simulink model "lookuptable"  (R2020a)
settings: Solver=FixedStepDiscrete  StartTime=0.0  StopTime=options.T_train  RelTol=1e-3
PreLoadFcn:
  | Ts = 0.1;
  | Plant = c2d(zpk([],[-1 -3 -5],1),Ts);
  | C0 = pid(1,1,1,'Ts',Ts,'IF','B','DF','B'); % define PID structure
  | C = pidtune(Plant,C0); % design PID
  | [Kp Ki Kd] = piddata(C); % obtain PID gains
  | FIS = sugfis;
  | FIS = addInput(FIS,[-10 10],'Name','E');
  | FIS = addMF(FIS,'E','gaussmf',[7 -10],'Name','Negative');
  | FIS = addMF(FIS,'E','gaussmf',[7 10],'Name','Positive');
  | FIS = addInput(FIS,[-10 10],'Name','CE');
  | FIS = addMF(FIS,'CE','gaussmf',[7 -10],'Name','Negative');
  | FIS = addMF(FIS,'CE','gaussmf',[7 10],'Name','Positive');
  | FIS = addOutput(FIS,[-20 20],'Name','u');
  | FIS = addMF(FIS,'u','constant',-20,'Name','Min');
  | FIS = addMF(FIS,'u','constant',0,'Name','Zero');
  | FIS = addMF(FIS,'u','constant',20,'Name','Max');
  | ruleList = [1 1 1 1 1;...   % Rule 1
  |             1 2 2 1 1;...   % Rule 2
  |             2 1 2 1 1;...   % Rule 3
  |             2 2 3 1 1];     % Rule 4
  | FIS = addRule(FIS,ruleList);GE = 10;
  | GCE = GE*(Kp-sqrt(Kp^2-4*Ki*Kd))/2/Ki;
  | GCU = Ki/GE;
  | GU = Kd/GCE;
  | Step = 1; % use 21 break points for both E and CE inputs
  | E = -10:Step:10;
  | CE = -10:Step:10;
  | N = length(E);
  | LookUpTableData = zeros(N);
  | for i=1:N
  |    for j=1:N
  |       % compute output u for each combination of break points
  |       LookUpTableData(i,j) = evalfis(FIS,[E(i) CE(j)]);
  |    end
  | end
undefined symbols (not defined in the file or in its folder): DiscIntNeverNeededParam, options
libraries: simulink x2, cstblocks x1
CloseFcn:
  | clear C E GCU Kd LookUpTableData Step j C0 FIS GE Ki N Ts ruleList CE GCE GU Kp Plant i
settings Model: FPTRunName=Active  Creator=The MathWorks, Inc.  LastModifiedBy=kekatos
settings DataIOCC: LimitDataPoints=on  SaveFormat=Array  ReturnWorkspaceOutputs=off
settings OptimizationCC: ExpressionDepthLimit=2147483647  LifeSpan=inf
settings DebuggingCC: UnderspecifiedInitializationDetection=Classic  MergeDetectMultiDrivingBlocksExec=none  SolverPrmCheckMsg=warning  FcnCallInpInsideContextMsg=warning  StateNameClashWarn=warning  SFUnexpectedBacktrackingDiag=warning  SFNoUnconditionalDefaultTransitionDiag=warning  SFExecutionAtInitializationDiag=none  ArithmeticOperatorsInVariantConditions=warning
settings HardwareCC: ProdBitPerPointer=32  ProdBitPerSizeT=32  ProdBitPerPtrDiffT=32  ProdLargestAtomicFloat=None  ProdIntDivRoundTo=Undefined  ProdEndianess=Unspecified  ProdWordSize=32  ProdHWDeviceType=32-bit Generic
settings ModelReferenceCC: PropagateSignalLabelsOutOfModel=off
settings SFSimCC: SimUseLocalCustomCode=off  CustomCodeUndefinedFunction=UseInterfaceOnly
settings RTWCC: RTWUseLocalCustomCode=off
settings CodeAppCC: StateflowObjectComments=on
settings GRTTargetCC: TargetLangStandard=C89/C90 (ANSI)  CombineOutputUpdateFcns=off  GRTInterface=on
settings ConfigComp: CovMetricSettings=dw  CovHtmlReporting=on  CovSaveCumulativeToWorkspaceVar=on  CovSaveSingleToWorkspaceVar=on  CovExternalEMLEnable=off

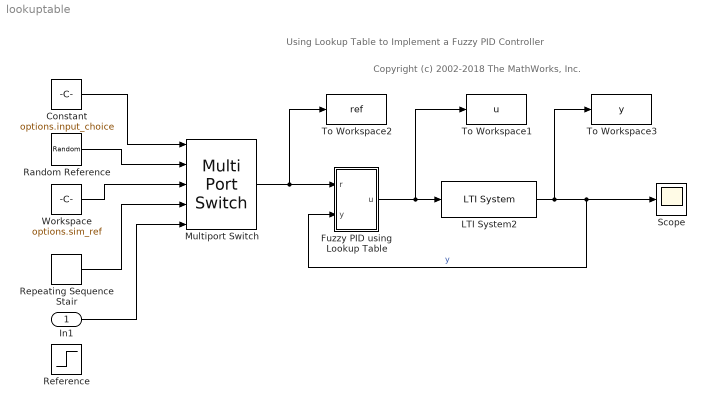
== system lookuptable ==
  note: Using Lookup Table to Implement a Fuzzy PID Controller
  note: Copyright (c) 2002-2018 The MathWorks, Inc.
  In1 : Inport
  Constant : Constant  Value=options.input_choice
  Fuzzy PID using Lookup Table : Subsystem
  LTI System2 : cstblocks/LTI System  sys=Plant  IC=[]
  Multiport Switch : MultiPortSwitch  Inputs=4
  Random Reference : UniformRandomNumber  Minimum=options.ref_min  Maximum=options.ref_max  Seed=randi(2^32,[1 ])  SampleTime=options.ref_Ts
  Reference : Step  SampleTime=0
  Repeating Sequence Stair : simulink/Sources/Repeating Sequence Stair  OutValues=options.sim_cov  tsamp=options.ref_Ts  OutMin=[]  OutMax=[]  OutDataTypeStr=double  OutputDataTypeScalingMode=double  OutDataType=fixdt(0,8)  ConRadixGroup=Best Precision: Vector-wise  OutScaling=2^-12
  Scope : Scope
  To Workspace1 : ToWorkspace  VariableName=u  SaveFormat=Structure With Time  SampleTime=options.dt
  To Workspace2 : ToWorkspace  VariableName=ref  SaveFormat=Structure With Time  SampleTime=options.dt
  To Workspace3 : ToWorkspace  VariableName=y  SaveFormat=Structure With Time  SampleTime=options.dt
  Workspace : Constant  Value=options.sim_ref
  wires:
  Fuzzy PID using Lookup Table/1(u) -> LTI System2/1, To Workspace1/1
  LTI System2/1 -> Scope/1, Fuzzy PID using Lookup Table/2(y), To Workspace3/1  "y"
  Workspace/1 -> Multiport Switch/3
  Random Reference/1 -> Multiport Switch/2
  Repeating Sequence Stair/1 -> Multiport Switch/4
  Constant/1 -> Multiport Switch/1
  In1/1 -> Multiport Switch/5
  Multiport Switch/1 -> To Workspace2/1, Fuzzy PID using Lookup Table/1(r)

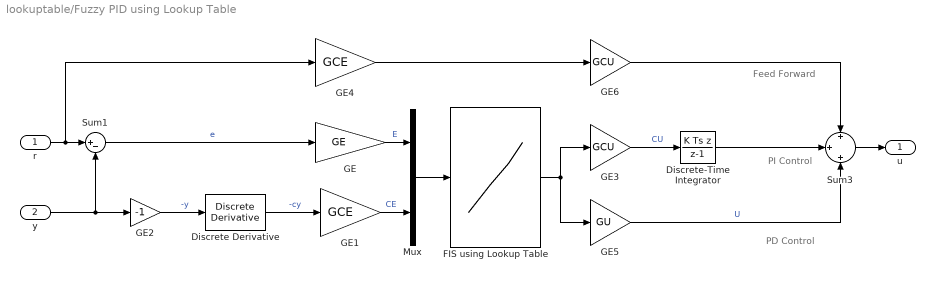
== system lookuptable/Fuzzy PID using Lookup Table ==
  note: PI Control
  note: PD Control
  note: Feed Forward
  r : Inport
  y : Inport  Port=2
  Discrete Derivative : simulink/Discrete/Discrete Derivative  gainval=1  ICPrevScaledInput=0.0  OutMin=[]  OutMax=[]  OutDataType=fixdt(1, 16)  OutScaling=2^-10  DoSatur=off
  Discrete-Time Integrator : DiscreteIntegrator  IntegratorMethod=Integration: Backward Euler  SampleTime=Ts  ICPrevOutput=DiscIntNeverNeededParam  ICPrevScaledInput=DiscIntNeverNeededParam
  FIS using Lookup Table : Lookup_n-D  BreakpointsForDimension1=E  BreakpointsForDimension2=CE  UseOneInputPortForAllInputData=on  Table=LookUpTableData  RndMeth=Simplest  InputSameDT=on
  GE : Gain  Gain=GE
  GE1 : Gain  Gain=GCE
  GE2 : Gain  Gain=-1
  GE3 : Gain  Gain=GCU
  GE4 : Gain  Gain=GCE
  GE5 : Gain  Gain=GU
  GE6 : Gain  Gain=GCU
  Mux : Mux  Inputs=2
  Sum1 : Sum  Inputs=|+-
  Sum3 : Sum  Inputs=+|+|+
  u : Outport  VectorParamsAs1DForOutWhenUnconnected=off
  wires:
  Sum1/1 -> GE/1  "e"
  Mux/1 -> FIS using Lookup Table/1
  GE/1 -> Mux/1  "E"
  GE1/1 -> Mux/2  "CE"
  FIS using Lookup Table/1 -> GE5/1, GE3/1
  GE3/1 -> Discrete-Time Integrator/1  "CU"
  GE5/1 -> Sum3/3  "U"
  GE2/1 -> Discrete Derivative/1  "-y"
  Discrete Derivative/1 -> GE1/1  "-cy"
  r/1 -> Sum1/1, GE4/1
  y/1 -> GE2/1, Sum1/2
  Discrete-Time Integrator/1 -> Sum3/2
  Sum3/1 -> u/1
  GE4/1 -> GE6/1
  GE6/1 -> Sum3/1
